simulink model "L4_5"  (R2023a)
settings: Solver=VariableStepAuto  StartTime=0.0  StopTime=100  RelTol=1e-8
undefined symbols (not defined in the file): k_i, k_p
settings Model: Creator=apere  LastModifiedBy=apere

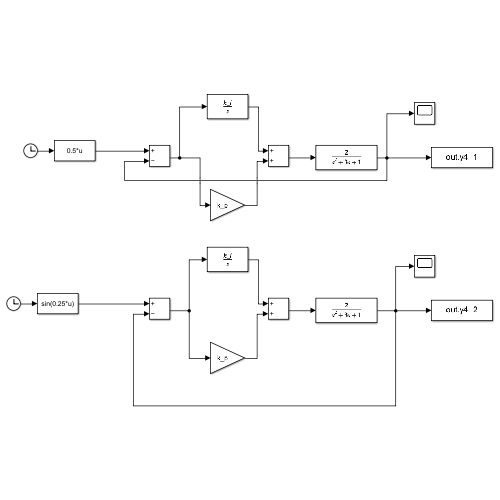
[thumbnail: Simulink's stored preview of the top-level diagram]
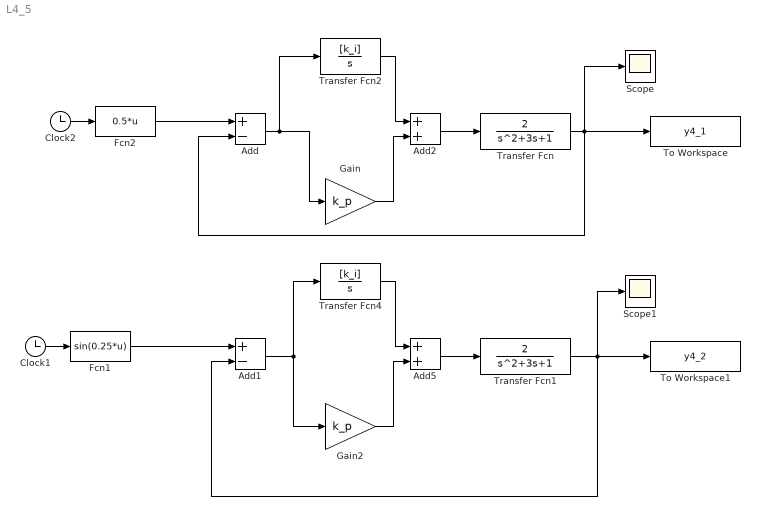
== system L4_5 ==
  Add : Sum  Inputs=+-
  Add1 : Sum  Inputs=+-
  Add2 : Sum
  Add5 : Sum
  Clock1 : Clock
  Clock2 : Clock
  Fcn1 : Fcn  Expr=sin(0.25*u)
  Fcn2 : Fcn  Expr=0.5*u
  Gain : Gain  Gain=k_p
  Gain2 : Gain  Gain=k_p
  Scope : Scope
  Scope1 : Scope
  To Workspace : ToWorkspace  VariableName=y4_1  SaveFormat=Timeseries  SampleTime=-1
  To Workspace1 : ToWorkspace  VariableName=y4_2  SaveFormat=Timeseries  SampleTime=-1
  Transfer Fcn : TransferFcn  Numerator=[2]  Denominator=[1 3 1]
  Transfer Fcn1 : TransferFcn  Numerator=[2]  Denominator=[1 3 1]
  Transfer Fcn2 : TransferFcn  Numerator=[k_i]  Denominator=[1 0]
  Transfer Fcn4 : TransferFcn  Numerator=[k_i]  Denominator=[1 0]
  wires:
  Transfer Fcn/1 -> Add/2, To Workspace/1, Scope/1
  Clock1/1 -> Fcn1/1
  Fcn2/1 -> Add/1
  Add/1 -> Gain/1, Transfer Fcn2/1
  Clock2/1 -> Fcn2/1
  Gain/1 -> Add2/2
  Transfer Fcn2/1 -> Add2/1
  Add2/1 -> Transfer Fcn/1
  Add1/1 -> Gain2/1, Transfer Fcn4/1
  Transfer Fcn4/1 -> Add5/1
  Add5/1 -> Transfer Fcn1/1
  Transfer Fcn1/1 -> Add1/2, To Workspace1/1, Scope1/1
  Gain2/1 -> Add5/2
  Fcn1/1 -> Add1/1
